simulink model "physicalModel"  (R2020b)
settings: Solver=ode3  StartTime=0.0  StopTime=10.0  FixedStep=Ts  RelTol=1e-3  EnableMultiTasking=on
values from neighbouring files (symbols this model uses):
  Vehicle = evalin('base','Vehicle')    [trimLinearize.m]
undefined symbols (not defined in the file or in its folder): Earth, init, WGS84
libraries: motorLib x4, shared6dof x1, aerolibtransform2 x1
settings Model: Creator=dbell44  LastModifiedBy=dbell44
settings DebuggingCC: BusObjectLabelMismatch=none

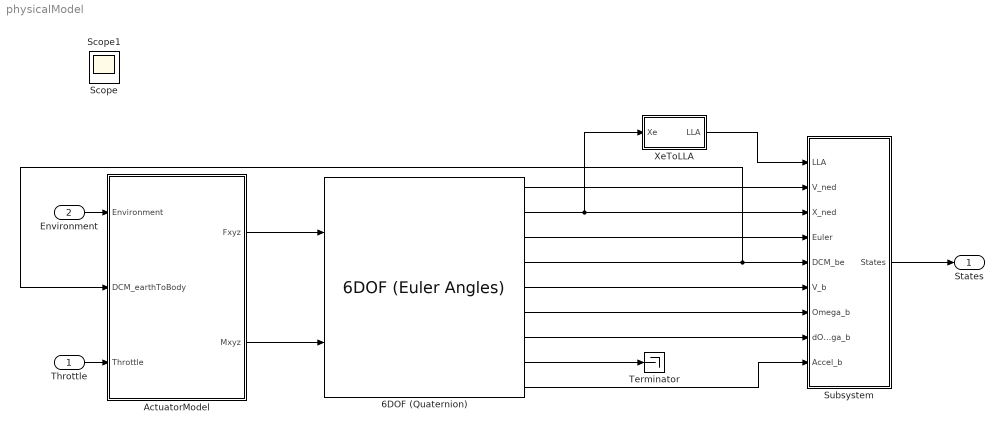
== system physicalModel ==
  Throttle : Inport  PortDimensions=[1 4]
  Environment : Inport  Port=2  OutDataTypeStr=Bus: EnvironmentBus  Interpolate=off
  6DOF (Quaternion) : shared6dof/6DOF (Euler Angles)  units=Metric (MKS)  mtype=Fixed  rep=Euler Angles  xme_0=init.posNED  Vm_0=init.vb  eul_0=init.euler  pm_0=init.angRates  mass_0=Vehicle.Airframe.mass  mass_e=0.5  mass_f=2.0  inertia=Vehicle.Airframe.inertia  inertia_e=eye(3)  inertia_f=2*eye(3)  k_quat=Vehicle.SixDOF.quatGain  vre_flag=on  abi_flag=on  aMode=aMode  xme_statename=''  Vm_statename=''  eul_statename=''  quat_statename=''  pm_statename=''  mass_statename=''
      settings: SourceProductBaseCode=AE,PW,MT,UV,VE,VP
  ActuatorModel : Subsystem  TreatAsAtomicUnit=on
  Subsystem : Subsystem
  Terminator : Terminator
  XeToLLA : Subsystem
  States : Outport  OutDataTypeStr=Bus: StatesBus
  Scope : Scope
  Scope1 : Scope
  wires:
  Environment/1 -> ActuatorModel/1(Environment)
  6DOF (Quaternion)/8 -> Terminator/1
  XeToLLA/1(LLA) -> Subsystem/1(LLA)
  6DOF (Quaternion)/1 -> Subsystem/2(V_ned)
  6DOF (Quaternion)/2 -> XeToLLA/1(Xe), Subsystem/3(X_ned)
  6DOF (Quaternion)/3 -> Subsystem/4(Euler)
  6DOF (Quaternion)/5 -> Subsystem/6(V_b)
  6DOF (Quaternion)/6 -> Subsystem/7(Omega_b)
  6DOF (Quaternion)/7 -> Subsystem/8(dOmega_b)
  6DOF (Quaternion)/9 -> Subsystem/9(Accel_b)
  6DOF (Quaternion)/4 -> ActuatorModel/2(DCM_earthToBody), Subsystem/5(DCM_be)
  Subsystem/1(States) -> States/1
  Throttle/1 -> ActuatorModel/3(Throttle)
  ActuatorModel/1(Fxyz) -> 6DOF (Quaternion)/1
  ActuatorModel/2(Mxyz) -> 6DOF (Quaternion)/2

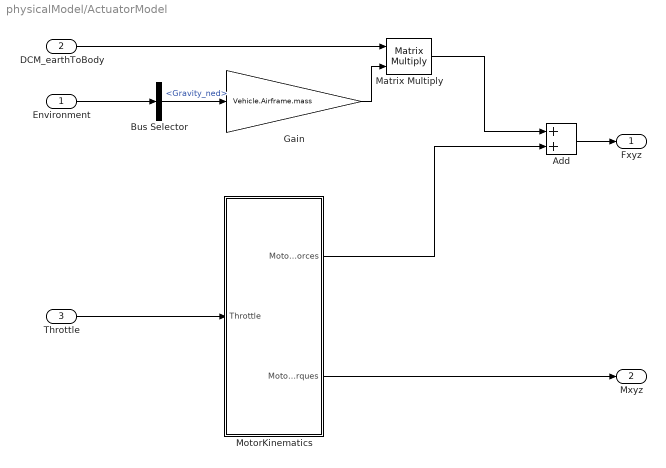
== system physicalModel/ActuatorModel ==
  Environment : Inport  OutDataTypeStr=Bus: EnvironmentBus
  DCM_earthToBody : Inport  Port=2
  Throttle : Inport  Port=3
  Add : Sum
  Bus Selector : BusSelector  OutputSignals=Gravity_ned
  Gain : Gain  Gain=Vehicle.Airframe.mass
  Matrix Multiply : Product  Multiplication=Matrix(*)
  MotorKinematics : Subsystem
  Fxyz : Outport
  Mxyz : Outport  Port=2
  wires:
  MotorKinematics/2(MotorTorques) -> Mxyz/1
  Environment/1 -> Bus Selector/1
  Bus Selector/1 -> Gain/1  "<Gravity_ned>"
  DCM_earthToBody/1 -> Matrix Multiply/1
  Gain/1 -> Matrix Multiply/2
  Matrix Multiply/1 -> Add/1
  Add/1 -> Fxyz/1
  Throttle/1 -> MotorKinematics/1(Throttle)
  MotorKinematics/1(MotorForces) -> Add/2

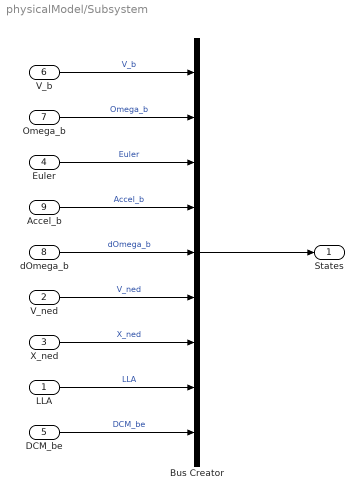
== system physicalModel/Subsystem ==
  LLA : Inport
  V_ned : Inport  Port=2
  X_ned : Inport  Port=3
  Euler : Inport  Port=4
  DCM_be : Inport  Port=5
  V_b : Inport  Port=6
  Omega_b : Inport  Port=7
  dOmega_b : Inport  Port=8
  Accel_b : Inport  Port=9
  Bus Creator : BusCreator  Inputs=9  OutDataTypeStr=Bus: StatesBus
      settings: InheritFromInputs=off
  States : Outport
  wires:
  LLA/1 -> Bus Creator/8  "LLA"
  V_ned/1 -> Bus Creator/6  "V_ned"
  X_ned/1 -> Bus Creator/7  "X_ned"
  Euler/1 -> Bus Creator/3  "Euler"
  DCM_be/1 -> Bus Creator/9  "DCM_be"
  V_b/1 -> Bus Creator/1  "V_b"
  Omega_b/1 -> Bus Creator/2  "Omega_b"
  dOmega_b/1 -> Bus Creator/5  "dOmega_b"
  Accel_b/1 -> Bus Creator/4  "Accel_b"
  Bus Creator/1 -> States/1

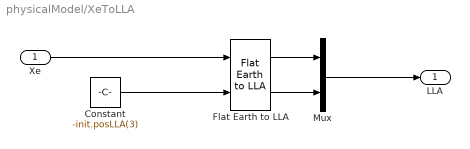
== system physicalModel/XeToLLA ==
  Xe : Inport
  Constant : Constant  Value=-init.posLLA(3)
  Flat Earth to LLA : aerolibtransform2/Flat Earth to LLA  units=Metric (MKS)  ptype=Earth (WGS84)  F=1/298.257223563  R=6378137  refPosPort=off  LL0=[0 10]  psi=0
  Mux : Mux  Inputs=2
  LLA : Outport
  wires:
  Xe/1 -> Flat Earth to LLA/1
  Mux/1 -> LLA/1
  Constant/1 -> Flat Earth to LLA/2
  Flat Earth to LLA/1 -> Mux/1
  Flat Earth to LLA/2 -> Mux/2

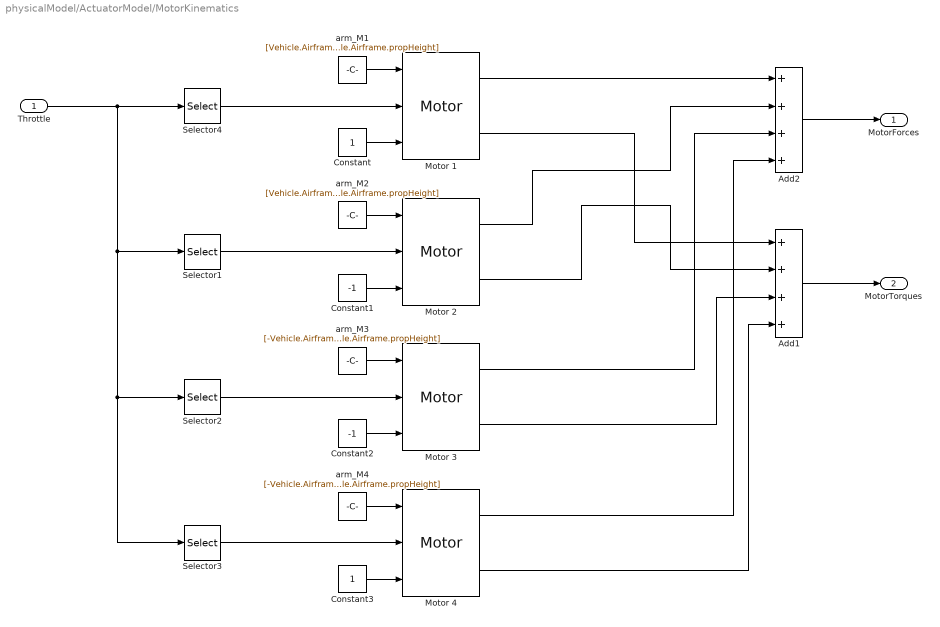
== system physicalModel/ActuatorModel/MotorKinematics ==
  Throttle : Inport
  Add1 : Sum  Inputs=++++
  Add2 : Sum  Inputs=++++
  Constant : Constant
  Constant1 : Constant  Value=-1
  Constant2 : Constant  Value=-1
  Constant3 : Constant
  Motor {1..4} (4 alike) : motorLib/Motor  SystemSampleTime=-1  VariantActivationTime=update diagram  Latency=0  AutoFrameSizeCalculation=off
  Selector1 : Selector  InputPortWidth=4  IndexOptions=Index vector (dialog)  Indices=2  OutputSizes=1
  Selector2 : Selector  InputPortWidth=4  IndexOptions=Index vector (dialog)  Indices=3  OutputSizes=1
  Selector3 : Selector  InputPortWidth=4  IndexOptions=Index vector (dialog)  Indices=4  OutputSizes=1
  Selector4 : Selector  InputPortWidth=4  IndexOptions=Index vector (dialog)  Indices=1  OutputSizes=1
  arm_M1 : Constant  Value=[Vehicle.Airframe.orthagPropDistance Vehicle.Airframe.orthagPropDistance Vehicle.Airframe.propHeight]
  arm_M2 : Constant  Value=[Vehicle.Airframe.orthagPropDistance -Vehicle.Airframe.orthagPropDistance Vehicle.Airframe.propHeight]
  arm_M3 : Constant  Value=[-Vehicle.Airframe.orthagPropDistance Vehicle.Airframe.orthagPropDistance Vehicle.Airframe.propHeight]
  arm_M4 : Constant  Value=[-Vehicle.Airframe.orthagPropDistance -Vehicle.Airframe.orthagPropDistance Vehicle.Airframe.propHeight]
  MotorForces : Outport
  MotorTorques : Outport  Port=2
  wires:
  Add1/1 -> MotorTorques/1
  Add2/1 -> MotorForces/1
  Motor 1/2 -> Add1/1
  Selector4/1 -> Motor 1/2
  Throttle/1 -> Selector3/1, Selector2/1, Selector1/1, Selector4/1
  arm_M2/1 -> Motor 2/1
  arm_M1/1 -> Motor 1/1
  Constant/1 -> Motor 1/3
  Motor 1/1 -> Add2/1
  Constant1/1 -> Motor 2/3
  arm_M3/1 -> Motor 3/1
  arm_M4/1 -> Motor 4/1
  Constant2/1 -> Motor 3/3
  Constant3/1 -> Motor 4/3
  Selector3/1 -> Motor 4/2
  Selector2/1 -> Motor 3/2
  Selector1/1 -> Motor 2/2
  Motor 2/1 -> Add2/2
  Motor 3/1 -> Add2/3
  Motor 4/1 -> Add2/4
  Motor 2/2 -> Add1/2
  Motor 3/2 -> Add1/3
  Motor 4/2 -> Add1/4
